simulink model "GraphicalFunction1"  (R2020a)
settings: Solver=FixedStepDiscrete  StartTime=0.0  StopTime=0.1  FixedStep=0.1  RelTol=1e-3  EnableMultiTasking=on
settings Model: Creator=bzhan  LastModifiedBy=bzhan
settings SolverCC: AutoInsertRateTranBlk=on
settings DataIOCC: LimitDataPoints=on
settings OptimizationCC: LifeSpan=inf
settings DebuggingCC: AllowSymbolicDim=off  SFUnexpectedBacktrackingDiag=warning  SFNoUnconditionalDefaultTransitionDiag=warning  SFExecutionAtInitializationDiag=none  ArithmeticOperatorsInVariantConditions=warning
settings SFSimCC: SimUseLocalCustomCode=off  CustomCodeUndefinedFunction=UseInterfaceOnly
settings RTWCC: RTWUseLocalCustomCode=off
settings CodeAppCC: StateflowObjectComments=on
settings GRTTargetCC: TargetLangStandard=C89/C90 (ANSI)
settings ConfigComp: CovMetricSettings=dw  CovHtmlReporting=on  CovSaveCumulativeToWorkspaceVar=on  CovSaveSingleToWorkspaceVar=on  CovShowResultsExplorer=off  CovExternalEMLEnable=off  CovSFcnEnable=off

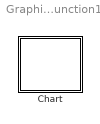
== system GraphicalFunction1 ==
  Chart : Stateflow chart  TreatAsAtomicUnit=on

== stateflow chart GraphicalFunction1/Chart ==
  state index=find [function]
    (junction 2) -> (junction 12) [order 3] : {index=i;}
    (default) -> (junction 2) : {i=1;}
    (junction 2) -> (junction 10) [order 2] : [i>N]
    (junction 10) -> (junction 12) : {index=-1;}
    (junction 2) -> (junction 5) [order 1] : [i<=N&&a(i)==0]
    (junction 6) -> (junction 2)
    (junction 5) -> (junction 6) : {i=i+1;}
  state A
    en: f("en_A")
  state B
    en: f("en_B")
  (default) -> A
  A -> B : [find()==3]
  data: index function_output; s function_input; a local =[0,0,1,2]; N local =4
  function f(s):
    | function f(s)
    |   fprintf(s+"\n");
